simulink subsystem "Gyroscope_SubSystem"  (R2020b)
settings: Solver=VariableStepAuto  StartTime=0.0  StopTime=10.0  RelTol=1e-3
undefined symbols (not defined in the file or in its folder): Ts
settings Model: Creator=umberto  LastModifiedBy=umberto

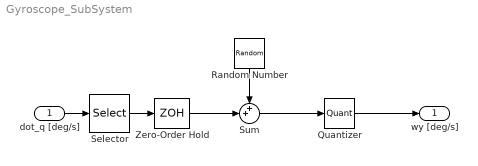
== system Gyroscope_SubSystem ==
  dot_q [deg/s] : Inport
  Quantizer : Quantizer  QuantizationInterval=sens.mpu.gyro.LSB2degs
  Random Number : RandomNumber  Variance=sens.mpu.gyro.noisevar  SampleTime=Ts
  Selector : Selector  InputPortWidth=2  IndexOptions=Index vector (dialog)  Indices=[2]  OutputSizes=1
  Sum : Sum  Inputs=++|
  Zero-Order Hold : ZeroOrderHold  SampleTime=Ts
  wy [deg/s] : Outport
  wires:
  Random Number/1 -> Sum/1
  Sum/1 -> Quantizer/1
  Zero-Order Hold/1 -> Sum/2
  Selector/1 -> Zero-Order Hold/1
  Quantizer/1 -> wy [deg/s]/1
  dot_q [deg/s]/1 -> Selector/1
